simulink model "LR_1_var15 (2)"  (R2020b)
settings: Solver=FixedStepAuto  StartTime=0.0  StopTime=10.0  FixedStep=0.001  RelTol=1e-3
libraries: simulink x7
settings Model: Creator=SIA  LastModifiedBy=SIA

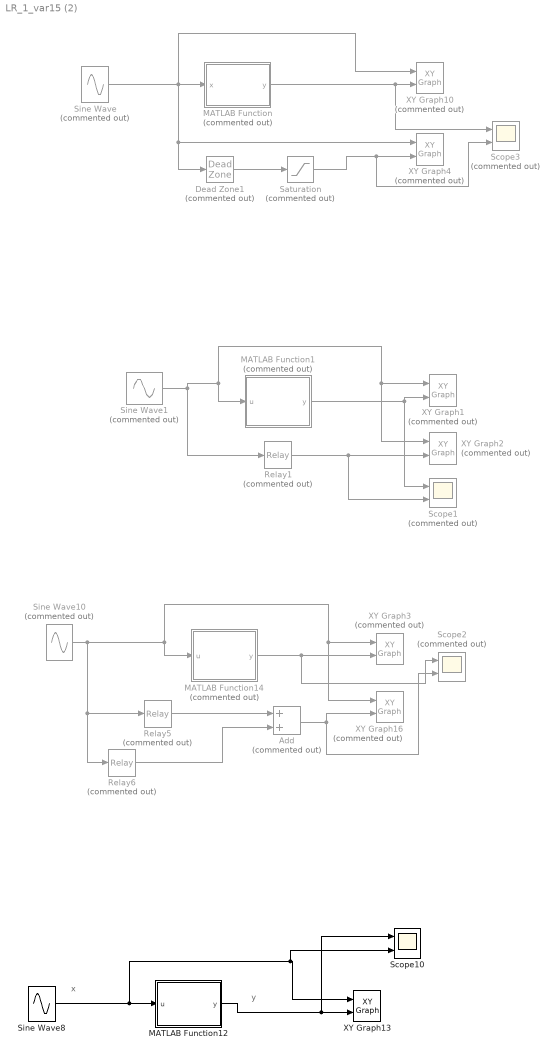
== system LR_1_var15 (2) ==
  note: x
  note: y
  Add : Sum  Commented=on
  Dead Zone1 : DeadZone  Commented=on  SaturateOnIntegerOverflow=on
  MATLAB Function : MATLAB Function  Commented=on  TreatAsAtomicUnit=on
  MATLAB Function1 : MATLAB Function  Commented=on  TreatAsAtomicUnit=on
  MATLAB Function12 : MATLAB Function  TreatAsAtomicUnit=on
  MATLAB Function14 : MATLAB Function  Commented=on  TreatAsAtomicUnit=on
  Relay1 : Relay  Commented=on  OnSwitchValue=0.6  OffSwitchValue=-0.6  OnOutputValue=2  OffOutputValue=-2
  Relay5 : Relay  Commented=on  OnSwitchValue=2  OffSwitchValue=1  OnOutputValue=3  OffOutputValue=-3
  Relay6 : Relay  Commented=on  OnSwitchValue=-1  OffSwitchValue=-2  OnOutputValue=3  OffOutputValue=-3
  Saturation : Saturate  Commented=on  UpperLimit=1  LowerLimit=-1
  Scope1 : Scope  Commented=on  NumInputPorts=2
  Scope10 : Scope  NumInputPorts=2
  Scope2 : Scope  Commented=on  NumInputPorts=2
  Scope3 : Scope  Commented=on  NumInputPorts=2
  Sine Wave : Sin  Commented=on  Amplitude=2  SampleTime=0
  Sine Wave1 : Sin  Commented=on  SampleTime=0
  Sine Wave10 : Sin  Commented=on  Amplitude=10  SampleTime=0
  Sine Wave8 : Sin  Amplitude=2.5  SampleTime=0
  XY Graph1 : simulink/Sinks/XY Graph  Commented=on  xmin=-4  xmax=4  ymin=-3  ymax=3  st=0.01
  XY Graph10 : simulink/Sinks/XY Graph  Commented=on  xmin=-2  xmax=2  ymin=-1.1  ymax=1.1  st=-1
  XY Graph13 : simulink/Sinks/XY Graph  xmin=-7  xmax=7  ymin=-8  ymax=8  st=0.001
  XY Graph16 : simulink/Sinks/XY Graph  Commented=on  xmin=-2  xmax=2  ymin=-6  ymax=6  st=0.001
  XY Graph2 : simulink/Sinks/XY Graph  Commented=on  xmin=-4  xmax=4  ymin=-3  ymax=3  st=0.01
  XY Graph3 : simulink/Sinks/XY Graph  Commented=on  xmin=-2  xmax=2  ymin=-6  ymax=6  st=0.001
  XY Graph4 : simulink/Sinks/XY Graph  Commented=on  xmin=-2  xmax=2  ymin=-1.1  ymax=1.1  st=-1
  wires:
  Sine Wave8/1 -> Scope10/2, XY Graph13/1, MATLAB Function12/1(u)
  MATLAB Function12/1(y) -> Scope10/1, XY Graph13/2
  MATLAB Function1/1(y) -> Scope1/1, XY Graph1/2
  Sine Wave1/1 -> MATLAB Function1/1(u), XY Graph2/1, XY Graph1/1, Relay1/1
  Relay1/1 -> Scope1/2, XY Graph2/2
  MATLAB Function14/1(y) -> Scope2/1, XY Graph3/2
  Relay5/1 -> Add/1
  Sine Wave10/1 -> MATLAB Function14/1(u), XY Graph3/1, XY Graph16/1, Relay5/1, Relay6/1
  Relay6/1 -> Add/2
  Add/1 -> Scope2/2, XY Graph16/2
  Saturation/1 -> Scope3/2, XY Graph4/2
  MATLAB Function/1(y) -> Scope3/1, XY Graph10/2
  Sine Wave/1 -> Dead Zone1/1, XY Graph4/1, XY Graph10/1, MATLAB Function/1(x)
  Dead Zone1/1 -> Saturation/1

== matlab function LR_1_var15 (2)/MATLAB Function1 ==
  data: u input; y output
function y = fcn(u)
persistent u2
c=2;
b=0.6;
y=-c;

if isempty(u2)
u2 = 0;
end

if u>u2
    if u>=b
        y=c;
    end
    if u<b
        y=-c;
    end
u2 = u;
end
if u<u2
    if u>-b
        y=c;
    end
    if u<=-b
        y=-c;
    end
u2 = u;
end

== matlab function LR_1_var15 (2)/MATLAB Function14 ==
  data: u input; y output
function y = fcn(u)
persistent u2
C=6;
b1=1;
b2 = 2;
y=-C;

if isempty(u2)
u2 = 0.1;
end

if u>u2
    if u>=b2
        y=C;
    end
    if (u>=-b1)&&(u<=b2)
        y=0;
    end
    if u<=-b1
        y=-C;
    end
u2 = u;
end
if u<u2
    if u>=b1
        y=C;
    end
    if (u>=-b2)&&(u<=b1)
        y=0;
    end
    if u<=-b2
        y=-C;
    end
u2 = u;
end

== matlab function LR_1_var15 (2)/MATLAB Function ==
  data: x input; y output
function y = fcn(x)
a=0.5;
M=1;
C=1.5;
k=M/(C-a);
if abs(x)<a
    y=0;
elseif (a<x)&&(x<C)
    y=k*(x-a);
elseif (a<-x)&&(-x<C)
    y=k*(x+a);
elseif x>C
    y=M;
else
    y=-M;
end

== matlab function LR_1_var15 (2)/MATLAB Function12 ==
  data: u input; y output
function y = fcn(u)
c=4;
b=2;
k = c/b;
y=0;

if u<=0
    y=-k*u;
end
if u>0
    y=k*u;
end

if u>=b
    y=-k*u+2*c;
end
end
